simulink model "Step2_Bimodal_NCM_ECM (1)"  (R2025b)
settings: Solver=VariableStepAuto  StartTime=0.0  StopTime=1800  RelTol=1e-3
values from neighbouring files (symbols this model uses):
  Cdl = (Qdl .* (Rct1 .^ (1 - n))) .^ (1 ./ n)    [Re_Step2_EC_fitting_with_EIS.m]
  ratios = 0:0.1:1    [Re_Step1_EIS_data_generation_noise.m]    (also in Re_Step2_EC_fitting_with_EIS.m = 0.0:0.1:1.0; Step2_EC_fitting_with_EIS.m = 0.0:0.1:1.0)
  Rct1 = (R*T) / (F*i0*S1)    [Re_Step1_EIS_data_generation_noise.m]    (also in Re_Step2_EC_fitting_with_EIS.m = fit_params_all(:, 4))
  Rct2 = (R*T) / (F*i0*S2)    [Re_Step1_EIS_data_generation_noise.m]    (also in Re_Step2_EC_fitting_with_EIS.m = fit_params_all(:, 7))
  Rs = 5    [Re_Step1_EIS_data_generation_noise.m]    (also in Re_Step2_EC_fitting_with_EIS.m = fit_params_all(:, 1))
  Rw1 = fit_params_all(:, 5)    [Re_Step2_EC_fitting_with_EIS.m]
  Rw2 = fit_params_all(:, 8)    [Re_Step2_EC_fitting_with_EIS.m]
libraries: nesl_utility x10, fl_lib x9, ee_lib x1
settings Model: Creator=ITBANK 510_02  LastModifiedBy=ITBANK 510_02
settings DebuggingCC: AlgebraicLoopMsg=none

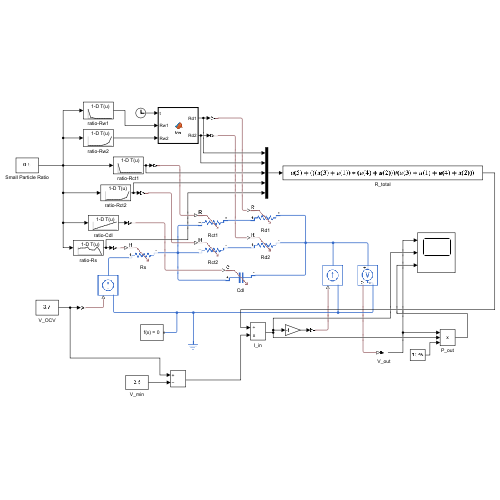
[thumbnail: Simulink's stored preview of the top-level diagram]
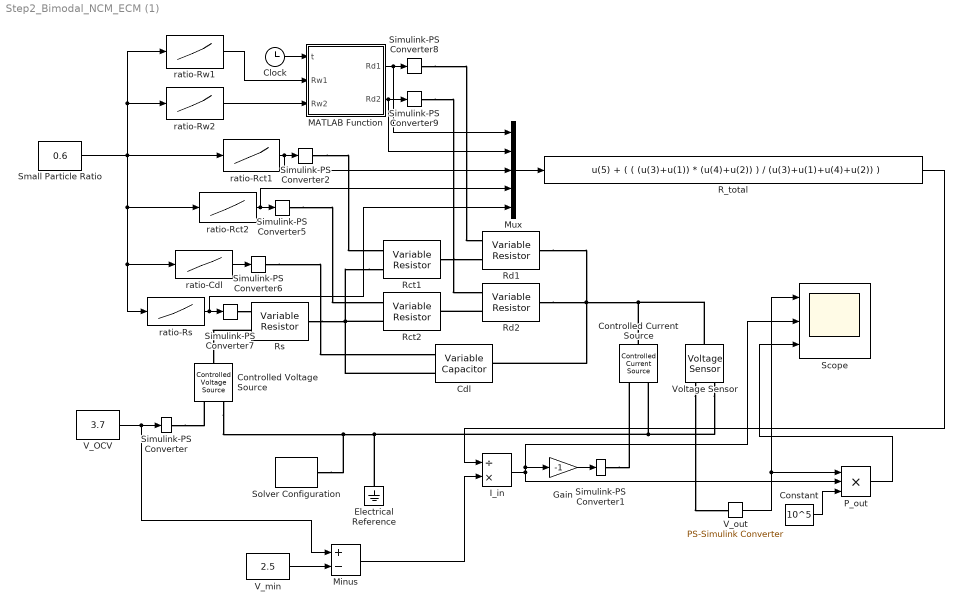
== system Step2_Bimodal_NCM_ECM (1) ==
  Cdl : ee_lib/Passive/Variable Capacitor  prm=2  Cmin=1e-9 F  r=1e-6 Ohm  v0=0 V  q0=0 C
      settings: InternalSimscapePortConfiguration="{\"Bottom\":[],\"Left\":[{\"id\":\"C\",\"label\":\"C\",\"type\":\"input\"},{\"id\":\"p\",\"label\":\"+\",\"type\":\"foundation.electrical.electrical\"}],\"Right\":[{\"id\":\"n\",\"label\":\"-\",\"type\":\"foundation.electrical.electrical\"}],\"Top\":[]}"
  Clock : Clock
  Constant : Constant  Value=10^5
  Controlled Current Source : fl_lib/Electrical/Electrical Sources/Controlled Current Source
  Controlled Voltage Source : fl_lib/Electrical/Electrical Sources/Controlled Voltage Source
  Electrical Reference : fl_lib/Electrical/Electrical Elements/Electrical Reference
  Gain : Gain  Gain=-1
  I_in : Product  Inputs=/*
  MATLAB Function : MATLAB Function  TreatAsAtomicUnit=on
  Minus : Sum  Inputs=+-
  Mux : Mux  Inputs=5
  P_out : Product  Inputs=3
  R_total : Fcn  Expr=u(5) + ( ( (u(3)+u(1)) * (u(4)+u(2)) ) / (u(3)+u(1)+u(4)+u(2)) )
  Rct1 : fl_lib/Electrical/Electrical Elements/Variable Resistor  Rmin=0 Ohm  thermalEnable=false  thermal_mass=1 J/K  i_specify=off  i_priority=None  i=0 A  i_nominal_specify=off  i_nominal_value=1  i_nominal_unit=A  v_specify=off  v_priority=None  v=0 V  v_nominal_specify=off  v_nominal_value=1  v_nominal_unit=V  T_specify=off  T_priority=None  T=300 K  T_nominal_specify=off  T_nominal_value=1  T_nominal_unit=K
  Rct2 : fl_lib/Electrical/Electrical Elements/Variable Resistor  Rmin=0 Ohm  thermalEnable=false  thermal_mass=1 J/K  i_specify=off  i_priority=None  i=0 A  i_nominal_specify=off  i_nominal_value=1  i_nominal_unit=A  v_specify=off  v_priority=None  v=0 V  v_nominal_specify=off  v_nominal_value=1  v_nominal_unit=V  T_specify=off  T_priority=None  T=300 K  T_nominal_specify=off  T_nominal_value=1  T_nominal_unit=K
  Rd1 : fl_lib/Electrical/Electrical Elements/Variable Resistor  Rmin=0 Ohm  thermalEnable=false  thermal_mass=1 J/K  i_specify=off  i_priority=None  i=0 A  i_nominal_specify=off  i_nominal_value=1  i_nominal_unit=A  v_specify=off  v_priority=None  v=0 V  v_nominal_specify=off  v_nominal_value=1  v_nominal_unit=V  T_specify=off  T_priority=None  T=300 K  T_nominal_specify=off  T_nominal_value=1  T_nominal_unit=K
  Rd2 : fl_lib/Electrical/Electrical Elements/Variable Resistor  Rmin=0 Ohm  thermalEnable=false  thermal_mass=1 J/K  i_specify=off  i_priority=None  i=0 A  i_nominal_specify=off  i_nominal_value=1  i_nominal_unit=A  v_specify=off  v_priority=None  v=0 V  v_nominal_specify=off  v_nominal_value=1  v_nominal_unit=V  T_specify=off  T_priority=None  T=300 K  T_nominal_specify=off  T_nominal_value=1  T_nominal_unit=K
  Rs : fl_lib/Electrical/Electrical Elements/Variable Resistor  Rmin=0 Ohm  thermalEnable=false  thermal_mass=1 J/K  i_specify=off  i_priority=None  i=0 A  i_nominal_specify=off  i_nominal_value=1  i_nominal_unit=A  v_specify=off  v_priority=None  v=0 V  v_nominal_specify=off  v_nominal_value=1  v_nominal_unit=V  T_specify=off  T_priority=None  T=300 K  T_nominal_specify=off  T_nominal_value=1  T_nominal_unit=K
  Scope : Scope  NumInputPorts=3
      settings: ActiveDisplayYMinimum=-2688.8627097390067  ActiveDisplayYMaximum=36221.29237886257
  Simulink-PS Converter{,1..2,5..9} (8 alike) : nesl_utility/Simulink-PS Converter  PhysicalDomain=network_engine_domain  SubClassName=ps_input  LeftPortType=input  RightPortType=output  PseudoPeriodic=off  Frequencies=[]  NoiseDistribution=none  NoiseParameters=[]  Unit=1  AffineConversion=off  FilteringAndDerivatives=provide  SimscapeFilterOrder=1  InputFilterTimeConstant=0.001  UdotUserProvided=0
  Small Particle Ratio : Constant  Value=0.6
  Solver Configuration : nesl_utility/Solver Configuration  PhysicalDomain=network_engine_domain  SubClassName=solver  LeftPortType=input  RightPortType=generic  Tones=[]  Harmonics=[]  SimulateNoise=off  Profile=off  UseLocalSampling=off  EnableSwitchedLinearOptims=on  FrequencyDomain=off  UseCCode=off  RelTol=0.001  AbsTol=0.001  MinStep=1e-09  ToWorkspace=off  RevertToSquareIcSolve=off  NumHomotopyIterations=100  PhasorMode=off  PhasorModeNumHarmonics=1  ConsistencySolver=NEWTON_XTOL_AFTER_FTOL  IndexReductionMethod=DerivativeReplacement  DoDC=off  ResidualTolerance=1e-09  ConsistencyTolSource=GLOBAL  ConsistencyAbsTol=0.001  ConsistencyRelTol=0.001  ConsistencyTolFactor=0.001  UseLocalSolver=off  LocalSolverChoice=NE_BACKWARD_EULER_ADVANCER  ResolveIndetEquations=on  FunctionEvalNumThread=1  LocalSolverSampleTime=0.001  DoFixedCost=off  MaxNonlinIter=3  MaxModeIter=2  ComputeImpulses=off  ImpulseIterations=2  LinearAlgebra=auto  LinearAlgebraNumThread=0  EquationFormulation=NE_TIME_EF  DelaysMemoryBudget=1024  AutomaticFiltering=on  FilteringTimeConstant=0.001  PartitionStorageMethod=AS_NEEDED  PartitionMemoryBudget=1024  PartitionMethod=ROBUST  MultibodyUseLocalSolver=off  MultibodyLocalSolverChoice=ODE1  MultibodyLocalSolverSampleTime=0.001
  V_OCV : Constant  Value=3.7
  V_min : Constant  Value=2.5
  V_out : nesl_utility/PS-Simulink Converter  PhysicalDomain=network_engine_domain  SubClassName=ps_output  LeftPortType=input  RightPortType=output  PseudoPeriodic=off  Frequencies=[]  VectorFormat=inherit  Unit=inherit  AffineConversion=off
  Voltage Sensor : fl_lib/Electrical/Electrical Sensors/Voltage Sensor
  ratio-Cdl : Lookup_n-D  NumberOfTableDimensions=1  LookupTableObject=EIS  BreakpointsForDimension1=ratios  Table=Cdl  InternalRulePriority=Speed  RndMeth=Simplest
  ratio-Rct1 : Lookup_n-D  NumberOfTableDimensions=1  LookupTableObject=EIS  BreakpointsForDimension1=ratios  Table=Rct1  InternalRulePriority=Speed  RndMeth=Simplest
  ratio-Rct2 : Lookup_n-D  NumberOfTableDimensions=1  LookupTableObject=EIS  BreakpointsForDimension1=ratios  Table=Rct2  InternalRulePriority=Speed  RndMeth=Simplest
  ratio-Rs : Lookup_n-D  NumberOfTableDimensions=1  LookupTableObject=EIS  BreakpointsForDimension1=ratios  Table=Rs  InternalRulePriority=Speed  RndMeth=Simplest
  ratio-Rw1 : Lookup_n-D  NumberOfTableDimensions=1  LookupTableObject=EIS  BreakpointsForDimension1=ratios  Table=Rw1  InternalRulePriority=Speed  RndMeth=Simplest
  ratio-Rw2 : Lookup_n-D  NumberOfTableDimensions=1  LookupTableObject=EIS  BreakpointsForDimension1=ratios  Table=Rw2  InternalRulePriority=Speed  RndMeth=Simplest
  wires:
  V_OCV/1 -> Minus/1, Simulink-PS Converter/1
  Small Particle Ratio/1 -> ratio-Rs/1, ratio-Cdl/1, ratio-Rct2/1, ratio-Rw1/1, ratio-Rw2/1, ratio-Rct1/1
  ratio-Rct1/1 -> Mux/3, Simulink-PS Converter2/1
  ratio-Rct2/1 -> Mux/4, Simulink-PS Converter5/1
  ratio-Cdl/1 -> Simulink-PS Converter6/1
  ratio-Rs/1 -> Mux/5, Simulink-PS Converter7/1
  MATLAB Function/1(Rd1) -> Mux/1, Simulink-PS Converter8/1
  Clock/1 -> MATLAB Function/1(t)
  ratio-Rw1/1 -> MATLAB Function/2(Rw1)
  ratio-Rw2/1 -> MATLAB Function/3(Rw2)
  MATLAB Function/2(Rd2) -> Mux/2, Simulink-PS Converter9/1
  Mux/1 -> R_total/1
  V_min/1 -> Minus/2
  I_in/1 -> Gain/1, Scope/2, P_out/2
  Minus/1 -> I_in/2
  R_total/1 -> I_in/1
  V_out/1 -> Scope/1, P_out/1
  P_out/1 -> Scope/3
  Gain/1 -> Simulink-PS Converter1/1
  Constant/1 -> P_out/3
  connections:
  Voltage Sensor/RConn2 -- Electrical Reference/LConn1 -- Controlled Voltage Source/RConn2 -- Solver Configuration/RConn1 -- Controlled Current Source/RConn2
  Rct1/LConn2 -- Rs/RConn1 -- Cdl/LConn2 -- Rct2/LConn2
  Simulink-PS Converter1/RConn1 -- Controlled Current Source/RConn1
  Voltage Sensor/RConn1 -- V_out/LConn1
  Simulink-PS Converter/RConn1 -- Controlled Voltage Source/RConn1
  Rs/LConn2 -- Controlled Voltage Source/LConn1
  Voltage Sensor/LConn1 -- Controlled Current Source/LConn1 -- Rd2/RConn1 -- Rd1/RConn1 -- Cdl/RConn1
  Simulink-PS Converter2/RConn1 -- Rct1/LConn1
  Simulink-PS Converter5/RConn1 -- Rct2/LConn1
  Simulink-PS Converter6/RConn1 -- Cdl/LConn1
  Simulink-PS Converter7/RConn1 -- Rs/LConn1
  Rd2/LConn2 -- Rct2/RConn1
  Rct1/RConn1 -- Rd1/LConn2
  Simulink-PS Converter8/RConn1 -- Rd1/LConn1
  Simulink-PS Converter9/RConn1 -- Rd2/LConn1

== matlab function Step2_Bimodal_NCM_ECM (1)/MATLAB Function ==
  data: t input; Rd1 output; Rw1 input; Rw2 input; Rd2 output
function [Rd1, Rd2] = fcn(t, Rw1, Rw2)
    % t: Clock 블록에서 들어오는 시뮬레이션 시간
    % Rw1, Rw2: 각 입자 브랜치의 Warburg 계수
    
    % 1. 고정 파라미터 설정
    tau1 = 400;      % 소립자 시상수
    tau2 = 1600;     % 대립자 시상수

    %% [Rd1 계산 - 소립자]
    % 소립자 전용 경계 설정
    t_short1 = 0.1 * tau1; % 40s
    t_long1  = 0.5 * tau1; % 200s

    if t < t_short1
        Rd1 = Rw1 * sqrt((4 * t) / (pi * tau1));
    elseif t > t_long1
        Rd1 = Rw1 * (t/tau1 + 1/3);
    else
        % 전이 구간 (40s ~ 200s) 선형 보간
        r1_at_short = Rw1 * sqrt((4 * t_short1) / (pi * tau1));
        r1_at_long  = Rw1 * (t_long1/tau1 + 1/3);
        Rd1 = r1_at_short + (r1_at_long - r1_at_short) * (t - t_short1) / (t_long1 - t_short1);
    end

    %% [Rd2 계산 - 대립자]
    % 대립자 전용 경계 설정
    t_short2 = 0.1 * tau2; % 160s
    t_long2  = 0.5 * tau2; % 800s

    if t < t_short2
        Rd2 = Rw2 * sqrt((4 * t) / (pi * tau2));
    elseif t > t_long2
        Rd2 = Rw2 * (t/tau2 + 1/3);
    else
        % 전이 구간 (160s ~ 800s) 선형 보간
        r2_at_short = Rw2 * sqrt((4 * t_short2) / (pi * tau2));
        r2_at_long  = Rw2 * (t_long2/tau2 + 1/3);
        Rd2 = r2_at_short + (r2_at_long - r2_at_short) * (t - t_short2) / (t_long2 - t_short2);
    end

    % 안전 장치
    if Rd1 < 0 || isnan(Rd1); Rd1 = 0; end
    if Rd2 < 0 || isnan(Rd2); Rd2 = 0; end
end
